simulink model "EXP04_task2b"  (R2020b)
settings: Solver=ode4  StartTime=0.0  StopTime=25  FixedStep=1e-3  RelTol=1e-3
values from neighbouring files (symbols this model uses):
  g = 9.81    [EXP04_Init.m]
  Kd = [kd,kd]    [EXP04_Init.m]
  Kp = [kp,kp]    [EXP04_Init.m]
  l1 = 1    [EXP04_Init.m]
  lc1 = l1/2    (= 0.5)    [EXP04_Init.m]
  lc2 = l2/2    (= 0.5)    [EXP04_Init.m]
  m1 = 10    [EXP04_Init.m]
  m2 = 7    [EXP04_Init.m]
  tau_down = -200    [EXP04_Init.m]
  tau_up = 200    [EXP04_Init.m]
undefined symbols (not defined in the file or in its folder): I1zz, I2zz
settings Model: Creator=baradaran  LastModifiedBy=jsol
settings DataIOCC: ReturnWorkspaceOutputs=off
settings DebuggingCC: ArithmeticOperatorsInVariantConditions=warning
settings SFSimCC: SimUseLocalCustomCode=off  CustomCodeUndefinedFunction=UseInterfaceOnly
settings RTWCC: RTWUseLocalCustomCode=off
settings CodeAppCC: StateflowObjectComments=on

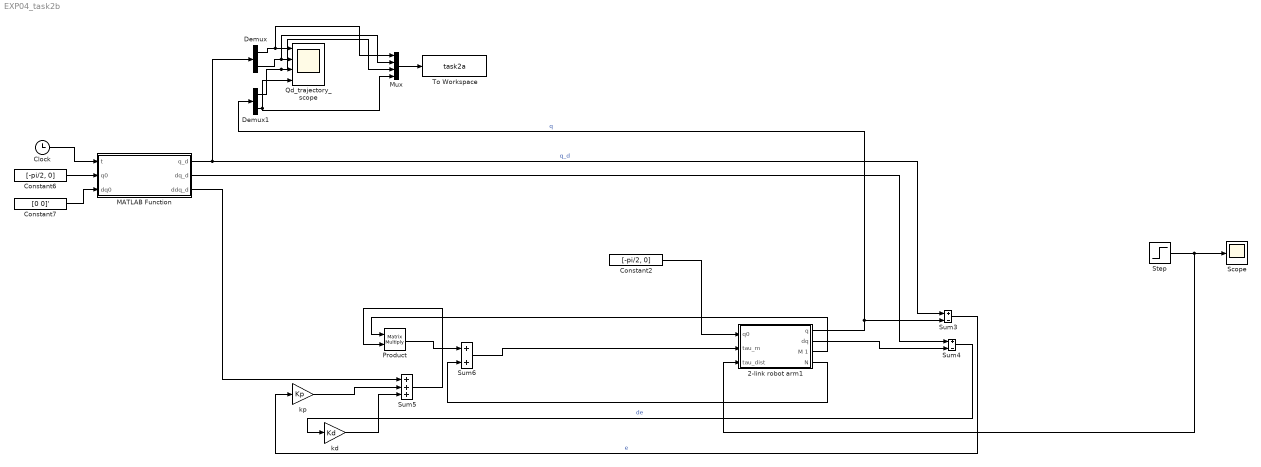
== system EXP04_task2b ==
  2-link robot arm1 : Subsystem
  Clock : Clock
  Constant2 : Constant  Value=[-pi/2, 0]
  Constant6 : Constant  Value=[-pi/2, 0]
  Constant7 : Constant  Value=[0 0]'
  Demux : Demux  Outputs=2
  Demux1 : Demux  Outputs=2
  MATLAB Function : MATLAB Function  TreatAsAtomicUnit=on
  Mux : Mux
  Product : Product  Multiplication=Matrix(*)
  Qd_trajectory_scope : Scope  NumInputPorts=4
  Scope : Scope
  Step : Step  Time=5  After=10  SampleTime=0
  Sum3 : Sum  Inputs=+-
  Sum4 : Sum  Inputs=+-
  Sum5 : Sum  Inputs=+++
  Sum6 : Sum
  To Workspace : ToWorkspace  VariableName=task2a  SaveFormat=Timeseries  SampleTime=-1
  kd : Gain  Gain=Kd
  kp : Gain  Gain=Kp
  wires:
  Constant6/1 -> MATLAB Function/2(q0)
  Clock/1 -> MATLAB Function/1(t)
  Constant7/1 -> MATLAB Function/3(dq0)
  Constant2/1 -> 2-link robot arm1/1(q0)
  MATLAB Function/1(q_d) -> Demux/1, Sum3/1  "q_d"
  MATLAB Function/2(dq_d) -> Sum4/1
  2-link robot arm1/1("q ") -> Demux1/1, Sum3/2  "q"
  2-link robot arm1/2("dq ") -> Sum4/2
  Sum3/1 -> kp/1  "e"
  Sum4/1 -> kd/1  "de"
  2-link robot arm1/3(M 1) -> Product/1
  kp/1 -> Sum5/2
  kd/1 -> Sum5/3
  MATLAB Function/3(ddq_d) -> Sum5/1
  Sum5/1 -> Product/2
  Product/1 -> Sum6/1
  2-link robot arm1/4("N ") -> Sum6/2
  Sum6/1 -> 2-link robot arm1/2(tau_m)
  Demux/1 -> Mux/1, Qd_trajectory_scope/1
  Demux/2 -> Mux/2, Qd_trajectory_scope/2
  Step/1 -> 2-link robot arm1/3(tau_dist), Scope/1
  Demux1/1 -> Mux/3, Qd_trajectory_scope/3
  Demux1/2 -> Qd_trajectory_scope/4, Mux/4
  Mux/1 -> To Workspace/1

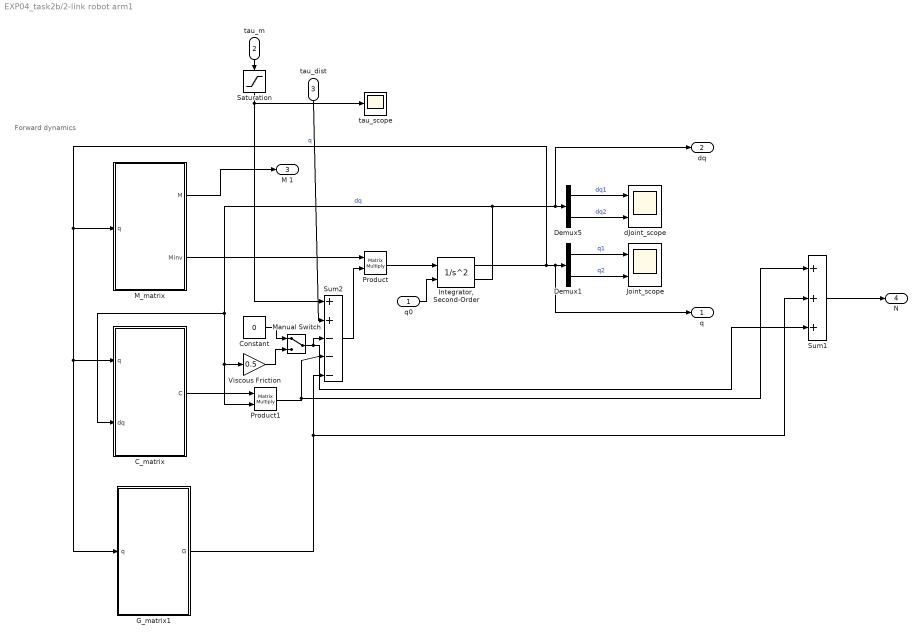
== system EXP04_task2b/2-link robot arm1 ==
  note: Forward dynamics
  q0 : Inport
  tau_m : Inport  Port=2
  tau_dist : Inport  Port=3
  C_matrix : MATLAB Function  TreatAsAtomicUnit=on
  Constant : Constant  Value=0
  Demux1 : Demux  Outputs=2
  Demux5 : Demux  Outputs=2
  G_matrix1 : MATLAB Function  TreatAsAtomicUnit=on
  "Integrator, Second-Order" : SecondOrderIntegrator  ICSourceX=external
  Joint_scope : Scope  NumInputPorts=2
  M_matrix : MATLAB Function  TreatAsAtomicUnit=on
  Manual Switch : ManualSwitch
  Product : Product  Multiplication=Matrix(*)
  Product1 : Product  Multiplication=Matrix(*)
  Saturation : Saturate  UpperLimit=tau_up  LowerLimit=tau_down
  Sum1 : Sum  Inputs=+++
  Sum2 : Sum  Inputs=++|---
  Viscous Friction : Gain  Gain=0.5
  dJoint_scope : Scope  NumInputPorts=2
  tau_scope : Scope
  "q " : Outport
  "dq " : Outport  Port=2
  M 1 : Outport  Port=3
  "N " : Outport  Port=4
  wires:
  Saturation/1 -> Sum2/1, tau_scope/1
  q0/1 -> "Integrator, Second-Order"/2
  tau_dist/1 -> Sum2/2
  tau_m/1 -> Saturation/1
  Manual Switch/1 -> Sum1/3, Sum2/3
  Product1/1 -> Sum1/1, Sum2/4
  G_matrix1/1(G) -> Sum1/2, Sum2/5
  Product/1 -> "Integrator, Second-Order"/1
  M_matrix/1(M) -> M 1/1
  Viscous Friction/1 -> Manual Switch/2
  Constant/1 -> Manual Switch/1
  Sum2/1 -> Product/2
  Demux5/2 -> dJoint_scope/2  "dq2"
  M_matrix/2(Minv) -> Product/1
  "Integrator, Second-Order"/1 -> Demux1/1, "q "/1, M_matrix/1(q), C_matrix/1(q), G_matrix1/1(q)  "q"
  C_matrix/1(C) -> Product1/1
  Demux5/1 -> dJoint_scope/1  "dq1"
  "Integrator, Second-Order"/2 -> Demux5/1, "dq "/1, Viscous Friction/1, Product1/2, C_matrix/2(dq)  "dq"
  Demux1/2 -> Joint_scope/2  "q2"
  Demux1/1 -> Joint_scope/1  "q1"
  Sum1/1 -> "N "/1

== matlab function EXP04_task2b/2-link robot arm1/C_matrix ==
  data: q input; C output; dq input; l1 parameter; lc2 parameter; m2 parameter
function C = C_matrix(q,dq, l1, lc2, m2)
%#codegen

%    This function was generated by the Symbolic Math Toolbox version 8.3.
%    05-Nov-2019 15:18:30
q1 = q(1);
q2 = q(2);
dq1 = dq(1);
dq2 = dq(2);
t2 = sin(q2);
C = reshape([-dq2.*l1.*lc2.*m2.*t2,dq1.*l1.*lc2.*m2.*t2,-l1.*lc2.*m2.*t2.*(dq1+dq2),0.0],[2,2]);

== matlab function EXP04_task2b/2-link robot arm1/G_matrix1 ==
  data: G output; q input; g parameter; l1 parameter; lc1 parameter; lc2 parameter; m1 parameter; m2 parameter
function G = G_matrix(q, g, l1, lc1, lc2, m1, m2)
%#codegen

%    This function was generated by the Symbolic Math Toolbox version 8.3.
%    05-Nov-2019 15:18:30
q1 = q(1);
q2 = q(2);
t2 = cos(q1);
t3 = q1+q2;
t4 = cos(t3);
G = [g.*m2.*(l1.*t2+lc2.*t4)+g.*lc1.*m1.*t2;g.*lc2.*m2.*t4];

== matlab function EXP04_task2b/2-link robot arm1/M_matrix ==
  data: M output; q input; I1zz parameter; I2zz parameter; l1 parameter; lc1 parameter; lc2 parameter; m1 parameter; m2 parameter; Minv output
function [M, Minv] = M_matrix(q, I1zz, I2zz, l1, lc1, lc2, m1, m2)
%#codegen

%    This function was generated by the Symbolic Math Toolbox version 8.3.
%    05-Nov-2019 15:18:29
q1 = q(1);
q2 = q(2);
t2 = cos(q2);
t3 = lc2.^2;
t4 = m2.*t3;
t5 = l1.*lc2.*m2.*t2;
t6 = I2zz+t4+t5;
M = reshape([I1zz+t5+t6+l1.^2.*m2+lc1.^2.*m1,t6,t6,I2zz+t4],[2,2]);
Minv = pinv(M);

== matlab function EXP04_task2b/MATLAB Function ==
  data: t input; q_d output; q0 input; dq0 input; dq_d output; ddq_d output
function [q_d, dq_d, ddq_d] = desired_traj(t,q0,dq0)
    A = 5*[1; 1];
    B = 5*[1; 1];
    w = 2*pi*1;

    q_d   = -A./w^2*sin(w*t) -B./(2*w)^2*cos(2*w*t) + dq0*t + q0;
    dq_d  = -A./w*cos(w*t) + B./(2*w)*sin(2*w*t) + dq0;
    ddq_d = A*sin(w*t) + B*cos(2*w*t);
end
